simulink model "sfbuilder_stats"  (Simulink 6.0)
settings: Solver=ode5  StartTime=0.0  StopTime=500  RelTol=1e-3
settings Model: Creator=The MathWorks Inc.  LastModifiedBy=batserve  ExtModeAutoUpdateStatusClock=off
settings DataIOCC: SignalLoggingName=sigsOut
settings DebuggingCC: CheckExecutionContextPreStartOutputMsg=on  CheckExecutionContextRuntimeOutputMsg=on  SolverPrmCheckMsg=none
settings HardwareCC: TargetUnknown=on

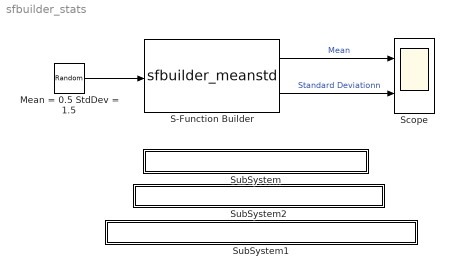
== system sfbuilder_stats ==
  Mean = 0.5 StdDev = 1.5 : RandomNumber  Mean=0.5  Variance=2.25  SampleTime=0.1
  S-Function Builder : S-Function  FunctionName=sfbuilder_meanstd  SFunctionModules=sfbuilder_meanstd_wrapper  WizardData=DataTag0  mask(S-Function Builder){}
      mask init:
      | val = [[.9  0.75 0.75 1 1 .9 .9 1]',[1 1 0.75 0.75 .9 .9 1 .9]'];
      | sys = get_param(gcb,'FunctionName');
      settings: CopyFcn=set_param(gcb,'LinkStatus','none')  OpenFcn=sfunctionwizard(gcbh)
      mask Display:
      | plot(val(:,1),val(:,2))
      | disp(sys)
      | port_label('input',1,'sig')
      | port_label('output',1,'Mean')
      | port_label('output',2,'stDeviation')
  Scope : Scope  NumInputPorts=2
      settings: TimeRange=500  YMin=0~0  YMax=2.5~2  SaveName=ScopeData2
  SubSystem : Subsystem  PropExecContextAcrossSSBoundary=on
      settings: AttributesFormatString=\n\n\n\n  OpenFcn=edit(fullfile(matlabroot,'simulink','src','sfbuilder_meanstd.c'))
      mask Display: disp('matlabroot\simulink\src\sfbuilder_meanstd.c');
  SubSystem1 : Subsystem  PropExecContextAcrossSSBoundary=on
      settings: AttributesFormatString=\n\n\n\n  OpenFcn=edit(fullfile(matlabroot,'toolbox','simulink','blocks','tlc_c','sfbuilder_meanstd.tlc'))
      mask Display: disp('matlabroot\toolbox\simulink\blocks\tlc_c\sfbuilder_meanstd.tlc');
  SubSystem2 : Subsystem  PropExecContextAcrossSSBoundary=on
      settings: AttributesFormatString=\n\n\n\n\n  OpenFcn=edit(fullfile(matlabroot,'simulink','src','sfbuilder_meanstd_wrapper.c'))
      mask Display: disp('matlabroot\simulink\src\sfbuilder_meanstd_wrapper.c');
  wires:
  Mean = 0.5 StdDev = 1.5/1 -> S-Function Builder/1
  S-Function Builder/1 -> Scope/1  "Mean"
  S-Function Builder/2 -> Scope/2  "Standard Deviationn"

== system sfbuilder_stats/SubSystem ==

== system sfbuilder_stats/SubSystem1 ==

== system sfbuilder_stats/SubSystem2 ==
